simulink model "verify_ThermalNodeTHB_mdl"  (R2016b)
settings: Solver=VariableStepAuto  StartTime=0.0  StopTime=3600  MaxStep=20  RelTol=1e-3  EnableMultiTasking=on
libraries: carnot x3
settings Model: Creator=drhf  LastModifiedBy=drhf
settings DataIOCC: LimitDataPoints=on  SaveFormat=Array  SignalLoggingSaveFormat=ModelDataLogs
settings OptimizationCC: ExpressionDepthLimit=2147483647  LifeSpan=inf
settings DebuggingCC: UnderspecifiedInitializationDetection=Classic  MergeDetectMultiDrivingBlocksExec=none  SolverPrmCheckMsg=warning  FcnCallInpInsideContextMsg=warning  StateNameClashWarn=warning  SFUnexpectedBacktrackingDiag=warning  SFNoUnconditionalDefaultTransitionDiag=warning  SFExecutionAtInitializationDiag=none
settings HardwareCC: ProdBitPerPointer=32  ProdBitPerSizeT=32  ProdBitPerPtrDiffT=32  ProdLargestAtomicFloat=None  ProdIntDivRoundTo=Undefined  ProdEndianess=Unspecified  ProdWordSize=32  ProdHWDeviceType=32-bit Generic
settings ModelReferenceCC: PropagateSignalLabelsOutOfModel=off
settings GRTTargetCC: TargetLangStandard=C89/C90 (ANSI)  GeneratePreprocessorConditionals=Disable all  CombineOutputUpdateFcns=off  GRTInterface=on
settings ConfigComp: CovMetricSettings=dw  CovHtmlReporting=on  CovSaveCumulativeToWorkspaceVar=on  CovSaveSingleToWorkspaceVar=on  CovExternalEMLEnable=off

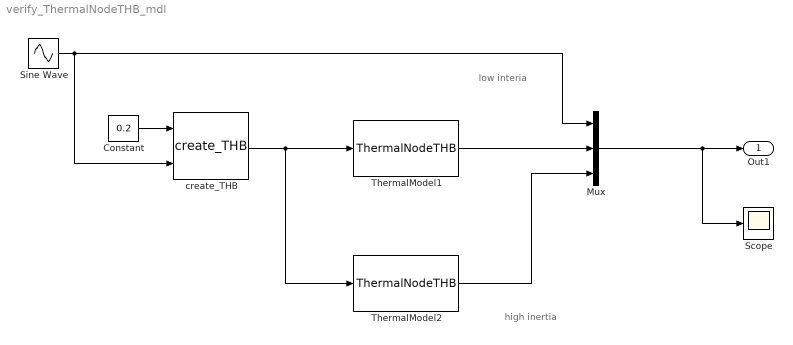
== system verify_ThermalNodeTHB_mdl ==
  note: low interia
  note: high inertia
  Constant : Constant  Value=0.2
  Mux : Mux  Inputs=3
  Scope : Scope
  Sine Wave : Sin  Amplitude=10  Bias=20  Frequency=2*pi/1800  SampleTime=0
  ThermalModel1 : carnot/Basic/Thermal_Models/ThermalNodeTHB  UA=0  mcp=40  Tini=20
  ThermalModel2 : carnot/Basic/Thermal_Models/ThermalNodeTHB  UA=10  mcp=10*4182  Tini=20
  create_THB : carnot/Source/Simple/create_THB  p=1e5  fluid=Water  mix=0  mix2=0  mix3=0  dia=0  hgt=0  mID=No Pressure Drop
  Out1 : Outport
  wires:
  Mux/1 -> Scope/1, Out1/1
  create_THB/1 -> ThermalModel2/1, ThermalModel1/1
  Constant/1 -> create_THB/1
  Sine Wave/1 -> create_THB/2, Mux/1
  ThermalModel1/1 -> Mux/2
  ThermalModel2/1 -> Mux/3
